simulink model "air_param_calculate"  (R2020b)
settings: Solver=VariableStepAuto  StartTime=0.0  StopTime=10.0  RelTol=1e-3
libraries: simulink x2
settings Model: Creator=Litao  LastModifiedBy=Litao

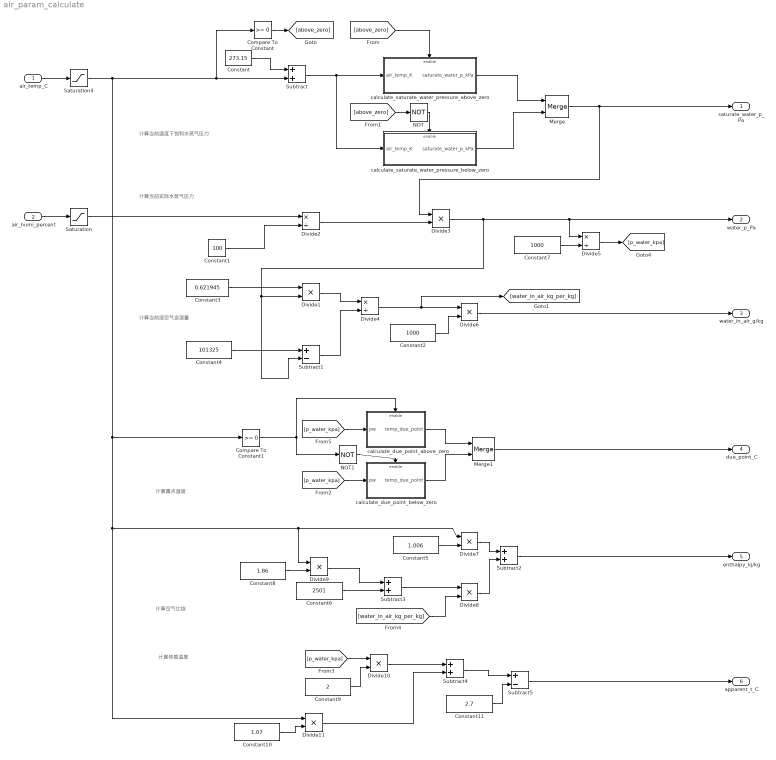
== system air_param_calculate ==
  note: 计算露点温度
  note: 计算当前湿空气含湿量
  note: 计算当前实际水蒸气压力
  note: 计算当前温度下饱和水蒸气压力
  note: 计算空气比焓
  note: 计算体感温度
  air_temp_C : Inport
  air_humi_percent : Inport  Port=2
  Compare To Constant : simulink/Logic and Bit Operations/Compare To Constant  relop=>=  const=0  OutDataTypeStr=boolean
  Compare To Constant1 : simulink/Logic and Bit Operations/Compare To Constant  relop=>=  const=0  OutDataTypeStr=boolean
  Constant : Constant  Value=273.15
  Constant1 : Constant  Value=100
  Constant10 : Constant  Value=1.07
  Constant11 : Constant  Value=2.7
  Constant2 : Constant  Value=1000
  Constant3 : Constant  Value=0.621945
  Constant4 : Constant  Value=101325
  Constant5 : Constant  Value=1.006
  Constant6 : Constant  Value=2501
  Constant7 : Constant  Value=1000
  Constant8 : Constant  Value=1.86
  Constant9 : Constant  Value=2
  Divide{1,3,6..11} (8 alike) : Product  Inputs=**
  Divide2 : Product  Inputs=*/
  Divide4 : Product  Inputs=*/
  Divide5 : Product  Inputs=*/
  Merge : Merge
  Merge1 : Merge
  NOT : Logic  Operator=NOT  IconShape=distinctive  AllPortsSameDT=off  OutDataTypeStr=boolean
  NOT1 : Logic  Operator=NOT  IconShape=distinctive  AllPortsSameDT=off  OutDataTypeStr=boolean
  Saturation : Saturate  UpperLimit=100.0  LowerLimit=0.0
  Saturation4 : Saturate  UpperLimit=60.0  LowerLimit=-30.0
  Subtract{,2..4} (4 alike) : Sum
  Subtract1 : Sum  Inputs=+-
  Subtract5 : Sum  Inputs=+-
  calculate_due_point_above_zero : Subsystem
  calculate_due_point_below_zero : Subsystem
  calculate_saturate_water_pressure_above_zero : Subsystem
  calculate_saturate_water_pressure_below_zero : Subsystem
  saturate_water_p_Pa : Outport
  water_p_Pa : Outport  Port=2
  water_in_air_g/kg : Outport  Port=3
  due_point_C : Outport  Port=4
  enthalpy_kj/kg : Outport  Port=5
  apparent_t_C : Outport  Port=6
  wires:
  air_humi_percent/1 -> Saturation/1
  Constant/1 -> Subtract/1
  Subtract/1 -> calculate_saturate_water_pressure_below_zero/1(air_temp_K), calculate_saturate_water_pressure_above_zero/1(air_temp_K)
  Compare To Constant/1 -> [above_zero]
  [above_zero] -> calculate_saturate_water_pressure_above_zero/Enable
  [above_zero] -> NOT/1
  NOT/1 -> calculate_saturate_water_pressure_below_zero/Enable
  calculate_saturate_water_pressure_above_zero/1(" saturate_water_p_kPa") -> Merge/1
  calculate_saturate_water_pressure_below_zero/1(" saturate_water_p_kPa") -> Merge/2
  Merge/1 -> saturate_water_p_Pa/1, Divide3/1
  Saturation/1 -> Divide2/1
  Constant1/1 -> Divide2/2
  Divide2/1 -> Divide3/2
  Divide1/1 -> Divide4/1
  Divide3/1 -> Divide5/1, water_p_Pa/1, Subtract1/2, Divide1/2
  Constant4/1 -> Subtract1/1
  Subtract1/1 -> Divide4/2
  Constant3/1 -> Divide1/1
  calculate_due_point_below_zero/1(" temp_due_point") -> Merge1/2
  NOT1/1 -> calculate_due_point_below_zero/Enable
  calculate_due_point_above_zero/1(" temp_due_point") -> Merge1/1
  [p_water_kpa] -> calculate_due_point_below_zero/1(pw)
  air_temp_C/1 -> Saturation4/1
  Compare To Constant1/1 -> calculate_due_point_above_zero/Enable, NOT1/1
  [p_water_kpa] -> calculate_due_point_above_zero/1(pw)
  Constant7/1 -> Divide5/2
  Divide5/1 -> [p_water_kpa]
  Merge1/1 -> due_point_C/1
  Divide4/1 -> [water_in_air_kg_per_kg], Divide6/1
  Constant2/1 -> Divide6/2
  Divide6/1 -> water_in_air_g/kg/1
  Constant5/1 -> Divide7/2
  Divide7/1 -> Subtract2/1
  Constant6/1 -> Subtract3/2
  Constant8/1 -> Divide9/2
  Divide9/1 -> Subtract3/1
  Subtract3/1 -> Divide8/1
  [water_in_air_kg_per_kg] -> Divide8/2
  Divide8/1 -> Subtract2/2
  Subtract2/1 -> enthalpy_kj/kg/1
  [p_water_kpa] -> Divide10/1
  Constant9/1 -> Divide10/2
  Constant10/1 -> Divide11/2
  Saturation4/1 -> Subtract/2, Compare To Constant/1, Divide11/1, Divide9/1, Divide7/1, Compare To Constant1/1
  Divide10/1 -> Subtract4/1
  Divide11/1 -> Subtract4/2
  Subtract4/1 -> Subtract5/1
  Constant11/1 -> Subtract5/2
  Subtract5/1 -> apparent_t_C/1

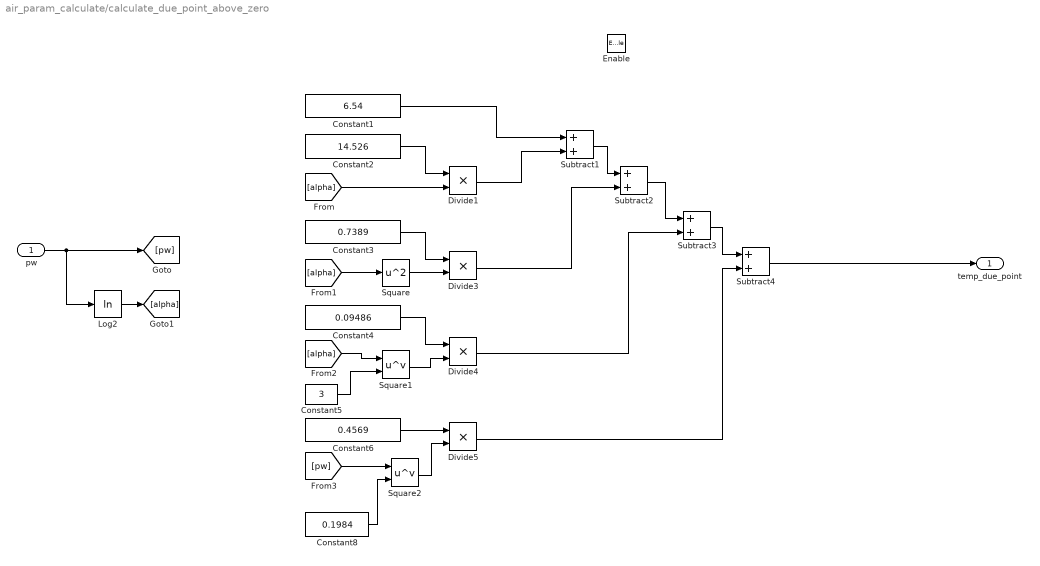
== system air_param_calculate/calculate_due_point_above_zero ==
  pw : Inport  OutDataTypeStr=double
  Enable : EnablePort
  Constant1 : Constant  Value=6.54  OutDataTypeStr=double
  Constant2 : Constant  Value=14.526  OutDataTypeStr=double
  Constant3 : Constant  Value=0.7389  OutDataTypeStr=double
  Constant4 : Constant  Value=0.09486  OutDataTypeStr=double
  Constant5 : Constant  Value=3  OutDataTypeStr=double
  Constant6 : Constant  Value=0.4569  OutDataTypeStr=double
  Constant8 : Constant  Value=0.1984  OutDataTypeStr=double
  Divide{1,3..5} (4 alike) : Product  Inputs=**
  Log2 : Math  Operator=log  OutputSignalType=real  SaturateOnIntegerOverflow=on
  Square : Math  Operator=square  SaturateOnIntegerOverflow=on
  Square1 : Math  Operator=pow  SaturateOnIntegerOverflow=on
  Square2 : Math  Operator=pow  SaturateOnIntegerOverflow=on
  Subtract{1..4} (4 alike) : Sum
  " temp_due_point" : Outport
  wires:
  pw/1 -> Log2/1, [pw]
  Constant1/1 -> Subtract1/1
  Constant2/1 -> Divide1/1
  [alpha] -> Divide1/2
  Divide1/1 -> Subtract1/2
  Divide3/1 -> Subtract2/2
  [alpha] -> Square/1
  Constant3/1 -> Divide3/1
  Square/1 -> Divide3/2
  Subtract1/1 -> Subtract2/1
  Square1/1 -> Divide4/2
  Constant4/1 -> Divide4/1
  [alpha] -> Square1/1
  Divide4/1 -> Subtract3/2
  Constant5/1 -> Square1/2
  Subtract2/1 -> Subtract3/1
  Constant6/1 -> Divide5/1
  Square2/1 -> Divide5/2
  Divide5/1 -> Subtract4/2
  Subtract3/1 -> Subtract4/1
  Subtract4/1 -> " temp_due_point"/1
  Log2/1 -> [alpha]
  [pw] -> Square2/1
  Constant8/1 -> Square2/2

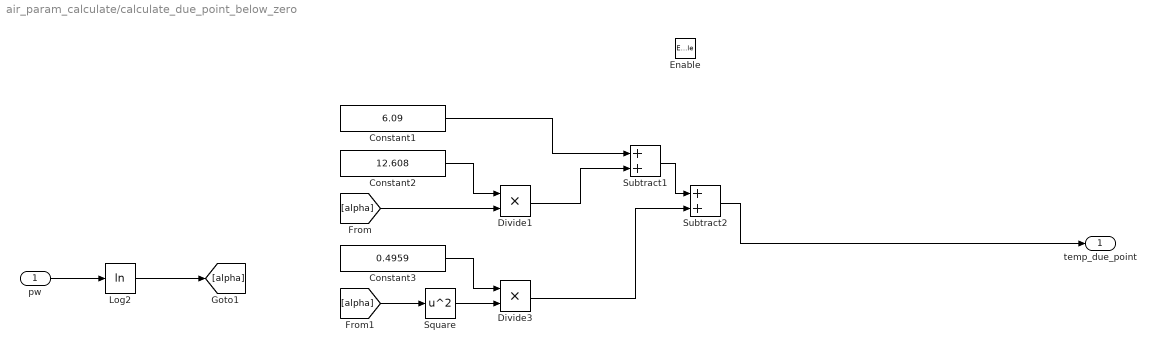
== system air_param_calculate/calculate_due_point_below_zero ==
  pw : Inport  OutDataTypeStr=double
  Enable : EnablePort
  Constant1 : Constant  Value=6.09  OutDataTypeStr=double
  Constant2 : Constant  Value=12.608  OutDataTypeStr=double
  Constant3 : Constant  Value=0.4959  OutDataTypeStr=double
  Divide1 : Product  Inputs=**
  Divide3 : Product  Inputs=**
  Log2 : Math  Operator=log  OutputSignalType=real  SaturateOnIntegerOverflow=on
  Square : Math  Operator=square  SaturateOnIntegerOverflow=on
  Subtract1 : Sum
  Subtract2 : Sum
  " temp_due_point" : Outport
  wires:
  Log2/1 -> [alpha]
  Subtract2/1 -> " temp_due_point"/1
  Subtract1/1 -> Subtract2/1
  Square/1 -> Divide3/2
  Constant3/1 -> Divide3/1
  [alpha] -> Square/1
  Divide3/1 -> Subtract2/2
  Divide1/1 -> Subtract1/2
  [alpha] -> Divide1/2
  Constant2/1 -> Divide1/1
  Constant1/1 -> Subtract1/1
  pw/1 -> Log2/1

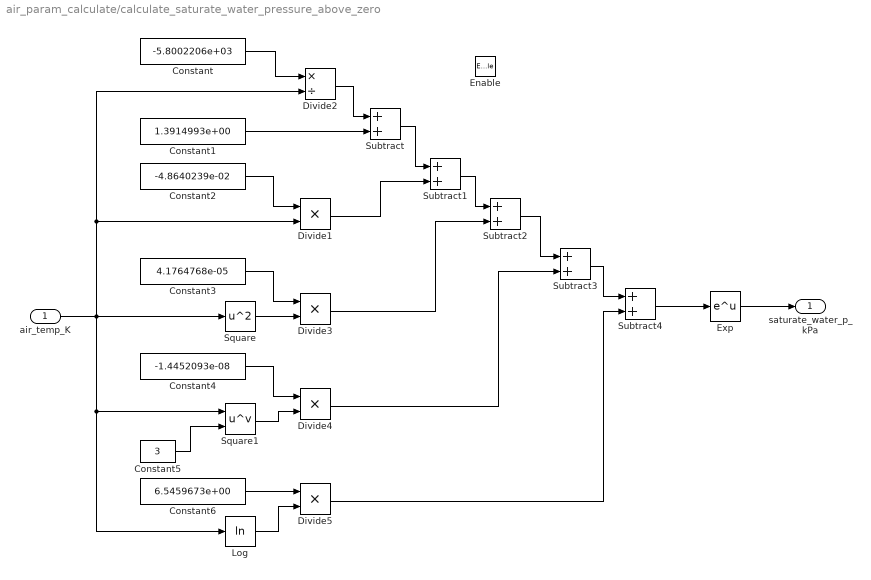
== system air_param_calculate/calculate_saturate_water_pressure_above_zero ==
  air_temp_K : Inport  OutDataTypeStr=double
  Enable : EnablePort
  Constant : Constant  Value=-5.8002206e+03  OutDataTypeStr=double
  Constant1 : Constant  Value=1.3914993e+00  OutDataTypeStr=double
  Constant2 : Constant  Value=-4.8640239e-02  OutDataTypeStr=double
  Constant3 : Constant  Value=4.1764768e-05  OutDataTypeStr=double
  Constant4 : Constant  Value=-1.4452093e-08  OutDataTypeStr=double
  Constant5 : Constant  Value=3  OutDataTypeStr=double
  Constant6 : Constant  Value=6.5459673e+00  OutDataTypeStr=double
  Divide{1,3..5} (4 alike) : Product  Inputs=**
  Divide2 : Product  Inputs=*/
  Exp : Math  SaturateOnIntegerOverflow=on
  Log : Math  Operator=log  OutputSignalType=real  SaturateOnIntegerOverflow=on
  Square : Math  Operator=square  SaturateOnIntegerOverflow=on
  Square1 : Math  Operator=pow  SaturateOnIntegerOverflow=on
  Subtract{,1..4} (5 alike) : Sum
  " saturate_water_p_kPa" : Outport  OutDataTypeStr=double
  wires:
  Constant2/1 -> Divide1/1
  Subtract4/1 -> Exp/1
  Log/1 -> Divide5/2
  Constant1/1 -> Subtract/2
  Constant4/1 -> Divide4/1
  Constant3/1 -> Divide3/1
  Subtract3/1 -> Subtract4/1
  Divide5/1 -> Subtract4/2
  Divide1/1 -> Subtract1/2
  Constant5/1 -> Square1/2
  Subtract1/1 -> Subtract2/1
  Divide3/1 -> Subtract2/2
  Square/1 -> Divide3/2
  Constant6/1 -> Divide5/1
  Divide4/1 -> Subtract3/2
  Square1/1 -> Divide4/2
  Subtract/1 -> Subtract1/1
  air_temp_K/1 -> Square/1, Square1/1, Log/1, Divide2/2, Divide1/2
  Divide2/1 -> Subtract/1
  Subtract2/1 -> Subtract3/1
  Exp/1 -> " saturate_water_p_kPa"/1
  Constant/1 -> Divide2/1

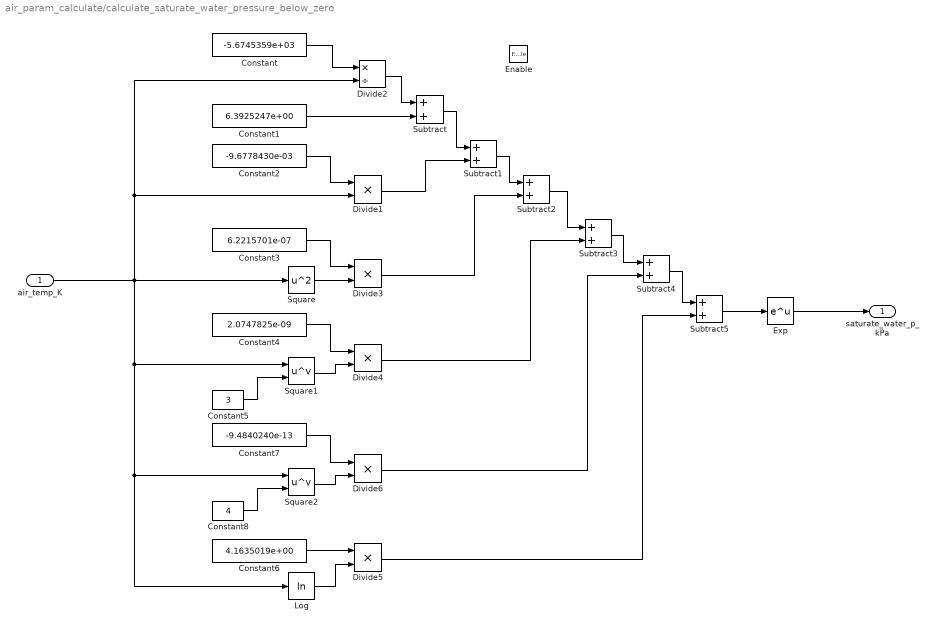
== system air_param_calculate/calculate_saturate_water_pressure_below_zero ==
  air_temp_K : Inport  OutDataTypeStr=double
  Enable : EnablePort
  Constant : Constant  Value=-5.6745359e+03  OutDataTypeStr=double
  Constant1 : Constant  Value=6.3925247e+00  OutDataTypeStr=double
  Constant2 : Constant  Value=-9.6778430e-03  OutDataTypeStr=double
  Constant3 : Constant  Value=6.2215701e-07  OutDataTypeStr=double
  Constant4 : Constant  Value=2.0747825e-09  OutDataTypeStr=double
  Constant5 : Constant  Value=3  OutDataTypeStr=double
  Constant6 : Constant  Value=4.1635019e+00  OutDataTypeStr=double
  Constant7 : Constant  Value=-9.4840240e-13  OutDataTypeStr=double
  Constant8 : Constant  Value=4  OutDataTypeStr=double
  Divide{1,3..6} (5 alike) : Product  Inputs=**
  Divide2 : Product  Inputs=*/
  Exp : Math  SaturateOnIntegerOverflow=on
  Log : Math  Operator=log  OutputSignalType=real  SaturateOnIntegerOverflow=on
  Square : Math  Operator=square  SaturateOnIntegerOverflow=on
  Square1 : Math  Operator=pow  SaturateOnIntegerOverflow=on
  Square2 : Math  Operator=pow  SaturateOnIntegerOverflow=on
  Subtract{,1..5} (6 alike) : Sum
  " saturate_water_p_kPa" : Outport  OutDataTypeStr=double
  wires:
  Constant/1 -> Divide2/1
  Divide2/1 -> Subtract/1
  Constant1/1 -> Subtract/2
  Subtract/1 -> Subtract1/1
  Constant2/1 -> Divide1/1
  Divide1/1 -> Subtract1/2
  Divide3/1 -> Subtract2/2
  Constant3/1 -> Divide3/1
  Square/1 -> Divide3/2
  Subtract1/1 -> Subtract2/1
  Square1/1 -> Divide4/2
  Constant4/1 -> Divide4/1
  Divide4/1 -> Subtract3/2
  Constant5/1 -> Square1/2
  Subtract2/1 -> Subtract3/1
  Constant6/1 -> Divide5/1
  air_temp_K/1 -> Log/1, Square2/1, Square1/1, Square/1, Divide1/2, Divide2/2
  Log/1 -> Divide5/2
  Subtract3/1 -> Subtract4/1
  Exp/1 -> " saturate_water_p_kPa"/1
  Constant8/1 -> Square2/2
  Constant7/1 -> Divide6/1
  Square2/1 -> Divide6/2
  Divide6/1 -> Subtract4/2
  Subtract4/1 -> Subtract5/1
  Subtract5/1 -> Exp/1
  Divide5/1 -> Subtract5/2
